simulink model "Buck_bode"  (R2023b)
settings: Solver=ode45  StartTime=0.0  StopTime=Tend*5/2  RelTol=1e-3  EnableMultiTasking=on
PreLoadFcn:
  | load('watertankdat')
values from neighbouring files (symbols this model uses):
  Cdc = 1e-4    (= 0.0001)    [main.m]
  D = 0.3    [main.m]
  L = 1e-3    (= 0.001)    [main.m]
  Ro = 1    [main.m]
  Tend = 0.1    [main.m]
  Ts = 1/Fs    (= 0.0001)    [main.m]
  Tsamp = 1/Fsamp    (= 1e-06)    [main.m]
  Vg = 100    [main.m]
libraries: spsSeriesRLCBranchLib x3, spsBuckConverterLib x1, spsCurrentMeasurementLib x1, spsDCVoltageSourceLib x1, spsVoltageMeasurementLib x1, slctrl_fre x1, simulink x1, sps_lib x1
settings Model: Creator=The MathWorks, Inc.  LastModifiedBy=baik3-ad
settings SolverCC: AlgebraicLoopSolver=TrustRegion  MaxZcPerStep=1
settings DataIOCC: LimitDataPoints=on  SaveFormat=Array  ReturnWorkspaceOutputs=off  SignalLoggingName=logsOut
settings OptimizationCC: ExpressionDepthLimit=2147483647  InitFltsAndDblsToZero=on  LifeSpan=inf
settings DebuggingCC: SaveWithParameterizedLinksMsg=none  UnderspecifiedInitializationDetection=Classic  MergeDetectMultiDrivingBlocksExec=none  SignalResolutionControl=TryResolveAllWithWarning  MultiTaskDSMMsg=warning  FcnCallInpInsideContextMsg=warning  UnconnectedInputMsg=warning  UnconnectedOutputMsg=warning  UnconnectedLineMsg=warning  AllowSymbolicDim=off  StateNameClashWarn=warning  SFUnexpectedBacktrackingDiag=warning  SFNoUnconditionalDefaultTransitionDiag=warning  SFExecutionAtInitializationDiag=none  ArithmeticOperatorsInVariantConditions=warning
settings HardwareCC: ProdBitPerPointer=32  ProdBitPerSizeT=32  ProdBitPerPtrDiffT=32  ProdLargestAtomicFloat=None  ProdIntDivRoundTo=Undefined  ProdEndianess=Unspecified  ProdWordSize=32  ProdHWDeviceType=Specified
settings ModelReferenceCC: EnableRefExpFcnMdlSchedulingChecks=on  PropagateSignalLabelsOutOfModel=off
settings SFSimCC: SimUseLocalCustomCode=off  CustomCodeUndefinedFunction=UseInterfaceOnly
settings RTWCC: RTWUseLocalCustomCode=off  DLArmComputeVersion=19.05
settings CodeAppCC: StateflowObjectComments=on
settings GRTTargetCC: TargetFcnLib=ansi_tfl_tmw.mat  TargetLangStandard=C89/C90 (ANSI)  CombineOutputUpdateFcns=off  GRTInterface=on
settings ConfigComp: CovMetricSettings=dw  CovSaveCumulativeToWorkspaceVar=on  CovSaveSingleToWorkspaceVar=on  CovExternalEMLEnable=off

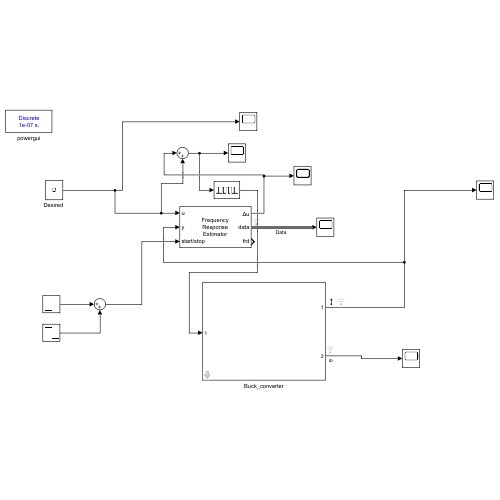
[thumbnail: Simulink's stored preview of the top-level diagram]
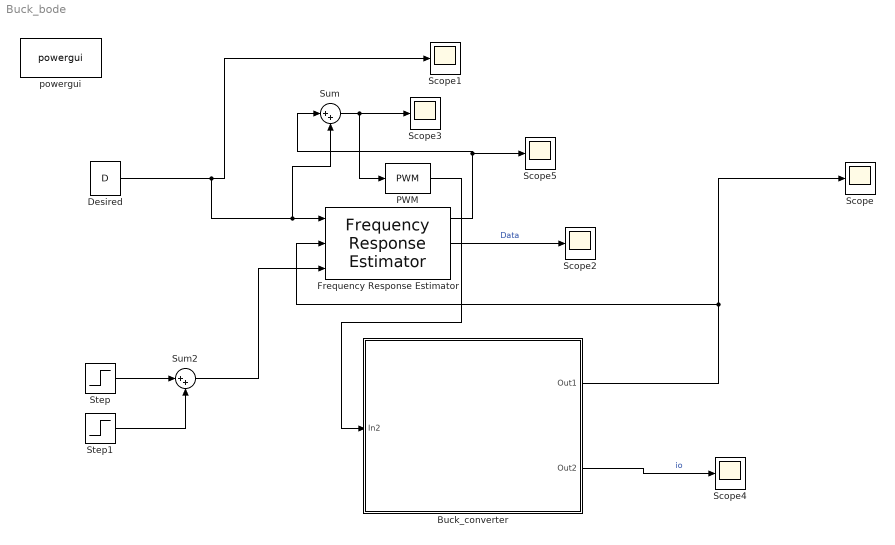
== system Buck_bode ==
  Buck_converter : Subsystem  mask{Vg=Vg, L=L, C=Cdc, R=Ro}
      mask prompts: Vg "Input voltage"; L "Output inductor"; C "Output capacitor"; R "Output resistor"
  "Desired " : Constant  Value=D
  Frequency Response Estimator : slctrl_fre/Frequency Response Estimator  DiscreteTs=Tsamp  OutputMode=perturbation only  BlockDataType=double  SineSource=Block parameters  Frequencies=ff  FreqUnits=Hz  Amplitudes=0.01  NumOfFreq=3  ExperimentMode=Sinestream  NumOfSetPeriod=5  NumOfEstPeriod=5  NumOfSlowestPeriod=3  NumOfPRBSPeriod=1  UseAutogenNumOfPRBSPeriod=off  PRBSSignalOrder=12  UseAutogenPRBSSignalOrder=off  EstimationMode=Online  UseBodePlot=on  BaselinePlant=[]  PlotRefreshFactor=100  UseExternalTs=off  BodePlotChoice=VariantBode  ExperimentChoice=VariantSS  OutputChoice=VariantDonly  CompiledTsChoice=InternalTs
      settings: LibrarySourceBlock=slctrlblks/Frequency Response Estimation/Frequency Response Estimator
  PWM : simulink/Discontinuities/PWM  DisableCoverage=on  Period=Ts  InitialDelay=0  DisallowZeroDutyCycle=off  RunAtFixedTimeIntervals=off  SampleTime=0.1
  Scope{,1..5} (6 alike) : Scope
  Step : Step  Time=Tend/2  SampleTime=0
  Step1 : Step  Time=0.5  After=-1  SampleTime=0
  Sum : Sum  Inputs=|++
  Sum2 : Sum  Inputs=|++
  powergui : sps_lib/powergui  Priority=1  SimulationMode=Discrete  SampleTime=Tsamp  frequency=60  Iterations=50  frequencyindice=0  Pbase=100e6  ErrMax=1e-4  UnitsV=kV  UnitsW=MW  buscounter=0  FunctionMessages=off  echomessages=off  EnableUseOfTLC=off  CurrentSourceSwitches=off  DisableSnubberDevices=off  DisableRonSwitches=off  DisableVfSwitches=off  DisplayEquations=off  AutomaticDiscreteSolvers=off  SolverType=Tustin/Backward Euler (TBE)  Interpol=off  ExternalGateDelay=off  methode=off  Ts=100  x0status=blocks  SPID=on  SwTol=0  HookPort=off  NonlinearTolerance=1e-4  nMaxIteration=100  ContinueOnMaxIteration=off  RestoreLinks=warning  ResistiveCurrentMeasurement=off  Frange=[0:2:500]  Ylog=off  Xlog=on  ShowGrid=off  save=off  variable=ZData  structure=0  ZoomFFT=off  StartTime=0.0  cycles=1  DisplayStyle=1  fundamental=60  FreqAxis=off  MaxFrequency=1000  frequencyindicesteady=1  RmsSteady=1  display=off
  wires:
  Buck_converter/1(Out1) -> Scope/1, Frequency Response Estimator/2
  "Desired "/1 -> Sum/2, Frequency Response Estimator/1, Scope1/1
  Frequency Response Estimator/2 -> Scope2/1  "Data"
  PWM/1 -> Buck_converter/1(In2)
  Sum2/1 -> Frequency Response Estimator/3
  Frequency Response Estimator/1 -> Sum/1, Scope5/1
  Sum/1 -> PWM/1, Scope3/1
  Step/1 -> Sum2/1
  Step1/1 -> Sum2/2
  Buck_converter/2(Out2) -> Scope4/1  "io"

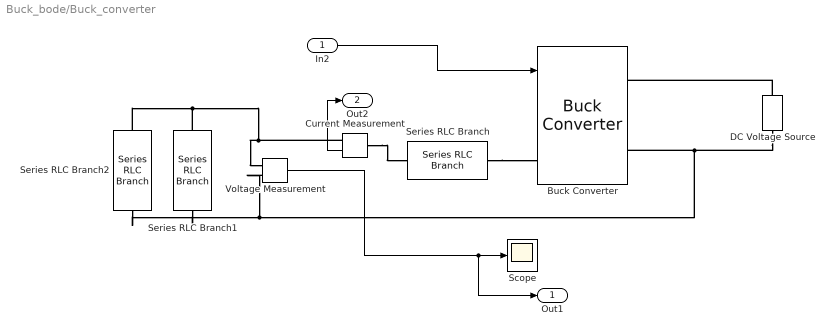
== system Buck_bode/Buck_converter ==
  In2 : Inport
  Buck Converter : spsBuckConverterLib/Buck Converter  ModelType=Switching devices  Ron=1e-3  Rs=1e8  Cs=inf  Vforward=[0,0]  Ron_Diode=1e-3  Rs_Diode=1e6  Cs_Diode=inf  Vf_Diode=1e-3  Rs_CurrentSource=inf  Ron_ACsource=1e-3
      settings: LibrarySourceBlock=sps_lib/Power Electronics/Buck Converter
  Current Measurement : spsCurrentMeasurementLib/Current Measurement  PhasorSimulation=off  OutputType=Complex  PSBequivalent=0
  DC Voltage Source : spsDCVoltageSourceLib/DC Voltage Source  Amplitude=Vg  Measurements=None
  Scope : Scope
  Series RLC Branch : spsSeriesRLCBranchLib/Series RLC Branch  LConnTagsString=__new0  RConnTagsString=__new0  BranchType=L  Resistance=1  Inductance=L  SetiL0=off  InitialCurrent=0  Capacitance=1e-6  Setx0=off  InitialVoltage=0  Measurements=None
  Series RLC Branch1 : spsSeriesRLCBranchLib/Series RLC Branch  LConnTagsString=__new0  RConnTagsString=__new0  BranchType=C  Resistance=1  Inductance=1e-3  SetiL0=off  InitialCurrent=0  Capacitance=C  Setx0=off  InitialVoltage=0  Measurements=None
  Series RLC Branch2 : spsSeriesRLCBranchLib/Series RLC Branch  LConnTagsString=__new0  RConnTagsString=__new0  BranchType=R  Resistance=R  Inductance=1e-3  SetiL0=off  InitialCurrent=0  Capacitance=1e-6  Setx0=off  InitialVoltage=0  Measurements=None
  Voltage Measurement : spsVoltageMeasurementLib/Voltage Measurement  PhasorSimulation=off  OutputType=Complex  PSBequivalent=0
  Out1 : Outport
  Out2 : Outport  Port=2
  wires:
  In2/1 -> Buck Converter/1
  Voltage Measurement/1 -> Out1/1, Scope/1
  Current Measurement/1 -> Out2/1
  connections:
  Voltage Measurement/LConn2 -- Series RLC Branch2/RConn1 -- Series RLC Branch1/RConn1 -- Buck Converter/RConn2 -- DC Voltage Source/LConn1
  Series RLC Branch2/LConn1 -- Series RLC Branch1/LConn1 -- Current Measurement/RConn1 -- Voltage Measurement/LConn1
  DC Voltage Source/RConn1 -- Buck Converter/RConn1
  Series RLC Branch/LConn1 -- Buck Converter/LConn1
  Current Measurement/LConn1 -- Series RLC Branch/RConn1
